simulink model "Longitudinal_Dynamics_Bicycle"  (R2020a)
settings: Solver=VariableStepAuto  StartTime=0.0  StopTime=10.0  MaxStep=0.2  RelTol=1e-3
settings Model: Creator=yafta  LastModifiedBy=yafta

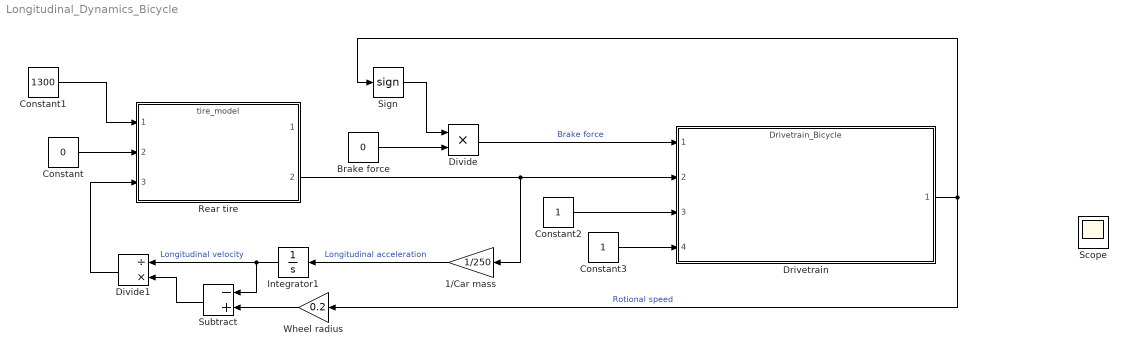
== system Longitudinal_Dynamics_Bicycle ==
  1/Car mass : Gain  Gain=1/250  OutDataTypeStr=double
  Brake force : Constant  Value=0  OutDataTypeStr=double
  Constant : Constant  Value=0  OutDataTypeStr=double
  Constant1 : Constant  Value=1300  OutDataTypeStr=double
  Constant2 : Constant  OutMin=[0]  OutMax=[5]  OutDataTypeStr=int8
  Constant3 : Constant
  Divide : Product  Inputs=**  OutDataTypeStr=double
  Divide1 : Product  Inputs=/*  OutDataTypeStr=double
  Drivetrain : ModelReference  ModelNameDialog=Drivetrain_Bicycle.slx  SimulationMode=Normal  ModelReferenceVersion=1.7
  Integrator1 : Integrator
  Rear tire : ModelReference  ModelNameDialog=tire_model.slx  SimulationMode=Normal  ModelReferenceVersion=1.8
  Scope : Scope
  Sign : Signum
  Subtract : Sum  Inputs=-+  AccumDataTypeStr=double
  Wheel radius : Gain  Gain=0.2  OutDataTypeStr=double
  wires:
  Drivetrain/1 -> Sign/1, Wheel radius/1  "Rotional speed"
  Wheel radius/1 -> Subtract/2
  Divide1/1 -> Rear tire/3
  Constant/1 -> Rear tire/2
  Integrator1/1 -> Divide1/1, Subtract/1  "Longitudinal velocity"
  1/Car mass/1 -> Integrator1/1  "Longitudinal acceleration"
  Subtract/1 -> Divide1/2
  Sign/1 -> Divide/1
  Constant1/1 -> Rear tire/1
  Brake force/1 -> Divide/2
  Divide/1 -> Drivetrain/1  "Brake force"
  Constant2/1 -> Drivetrain/3
  Rear tire/2 -> 1/Car mass/1, Drivetrain/2
  Constant3/1 -> Drivetrain/4
